simulink model "lab05par01"  (R2015a)
settings: Solver=ode45  StartTime=0.0  StopTime=10.0  RelTol=1e-3
settings Model: Creator=dg  LastModifiedBy=dg

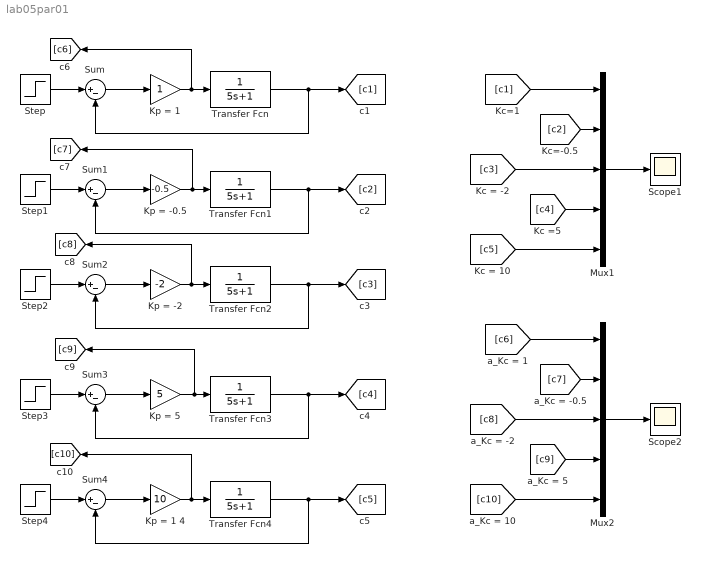
== system lab05par01 ==
  Kp = -0.5 : Gain  Gain=-0.5
  Kp = -2 : Gain  Gain=-2
  "Kp = 1 " : Gain
  Kp = 1 4 : Gain  Gain=10
  Kp = 5 : Gain  Gain=5
  Mux1 : Mux  Inputs=5
  Mux2 : Mux  Inputs=5
  Scope1 : Scope
      settings: ShowLegends=on  YMin=-1  YMax=1.5
  Scope2 : Scope
      settings: ShowLegends=on  YMax=10
  Step{,1..4} (5 alike) : Step  Time=0  SampleTime=0
  Sum{,1..4} (5 alike) : Sum  Inputs=|+-
  Transfer Fcn{,1..4} (5 alike) : TransferFcn  Denominator=[5 1]
  wires:
  Step/1 -> Sum/1
  Sum/1 -> "Kp = 1 "/1
  "Kp = 1 "/1 -> [c6], Transfer Fcn/1
  Transfer Fcn/1 -> Sum/2, [c1]
  Step1/1 -> Sum1/1
  Sum1/1 -> Kp = -0.5/1
  Kp = -0.5/1 -> [c7], Transfer Fcn1/1
  Transfer Fcn1/1 -> Sum1/2, [c2]
  Step2/1 -> Sum2/1
  Sum2/1 -> Kp = -2/1
  Kp = -2/1 -> [c8], Transfer Fcn2/1
  Transfer Fcn2/1 -> Sum2/2, [c3]
  Step3/1 -> Sum3/1
  Sum3/1 -> Kp = 5/1
  Kp = 5/1 -> [c9], Transfer Fcn3/1
  Transfer Fcn3/1 -> Sum3/2, [c4]
  Step4/1 -> Sum4/1
  Sum4/1 -> Kp = 1 4/1
  Kp = 1 4/1 -> [c10], Transfer Fcn4/1
  Transfer Fcn4/1 -> Sum4/2, [c5]
  Mux1/1 -> Scope1/1
  [c1] -> Mux1/1
  [c2] -> Mux1/2
  [c3] -> Mux1/3
  [c4] -> Mux1/4
  [c5] -> Mux1/5
  Mux2/1 -> Scope2/1
  [c6] -> Mux2/1
  [c7] -> Mux2/2
  [c8] -> Mux2/3
  [c9] -> Mux2/4
  [c10] -> Mux2/5
